simulink model "system"  (R2015a)
settings: Solver=ode45  StartTime=0.0  StopTime=10.0  RelTol=1e-3
values from neighbouring files (symbols this model uses):
  g = 9.81    [run_sim.m]    (also in run_sim_auto.m; run_sim_test.m; run_sim_test4.m; run_sim_v2.m)
  m = 210    [run_sim_auto.m]    (also in run_sim_test4.m = 150; sim_testing.m; wrkspc_no_1.mat; wrkspc_no_10.mat)
  rho_air = 1.225    [run_sim.m]    (also in run_sim_auto.m; run_sim_test.m; run_sim_test4.m; run_sim_v2.m)
undefined symbols (not defined in the file or in its folder): a, crr
libraries: simulink x1
settings Model: Creator=marco  LastModifiedBy=marco

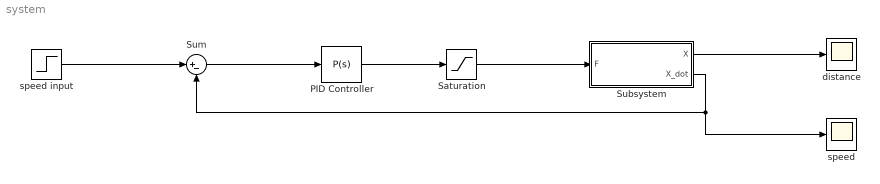
== system system ==
  PID Controller : simulink/Continuous/PID Controller  Controller=P  TimeDomain=Continuous-time  SampleTime=-1  IntegratorMethod=Forward Euler  FilterMethod=Forward Euler  Form=Parallel  UseFilter=on  ControllerParametersSource=internal  P=1  I=0  D=0  N=100  InitialConditionSource=internal  InitialConditionForIntegrator=0  InitialConditionForFilter=0  ExternalReset=none  LimitOutput=off  UpperSaturationLimit=inf  LowerSaturationLimit=-inf  LinearizeAsGain=on  AntiWindupMode=none  Kb=1  TrackingMode=off  Kt=1  PParamMin=[]  PParamMax=[]  IParamMin=[]  IParamMax=[]  DParamMin=[]  DParamMax=[]  NParamMin=[]  NParamMax=[]  KbParamMin=[]  KbParamMax=[]  KtParamMin=[]  KtParamMax=[]  POutMin=[]  POutMax=[]  IOutMin=[]  IOutMax=[]  DOutMin=[]  DOutMax=[]  NOutMin=[]  NOutMax=[]  KbOutMin=[]  KbOutMax=[]  KtOutMin=[]  KtOutMax=[]  IntegratorOutMin=[]  IntegratorOutMax=[]  FilterOutMin=[]  FilterOutMax=[]  SumOutMin=[]  SumOutMax=[]  SumI1OutMin=[]  SumI1OutMax=[]  SumI2OutMin=[]  SumI2OutMax=[]  SumI3OutMin=[]  SumI3OutMax=[]  SumDOutMin=[]  SumDOutMax=[]  SaturationOutMin=[]  SaturationOutMax=[]  IntegratorContinuousStateAttributes=''  IntegratorStateMustResolveToSignalObject=off  IntegratorRTWStateStorageClass=Auto  FilterContinuousStateAttributes=''  FilterStateMustResolveToSignalObject=off  FilterRTWStateStorageClass=Auto  DifferentiatorICPrevScaledInput=0  DifferentiatorOutMin=[]  DifferentiatorOutMax=[]
  Saturation : Saturate
  Subsystem : Subsystem
  Sum : Sum  Inputs=|+-
  distance : Scope
  speed : Scope
  speed input : Step  Before=1  SampleTime=0
  wires:
  Saturation/1 -> Subsystem/1(F)
  PID Controller/1 -> Saturation/1
  Sum/1 -> PID Controller/1
  Subsystem/2(X_dot) -> speed/1, Sum/2
  Subsystem/1(X) -> distance/1
  speed input/1 -> Sum/1

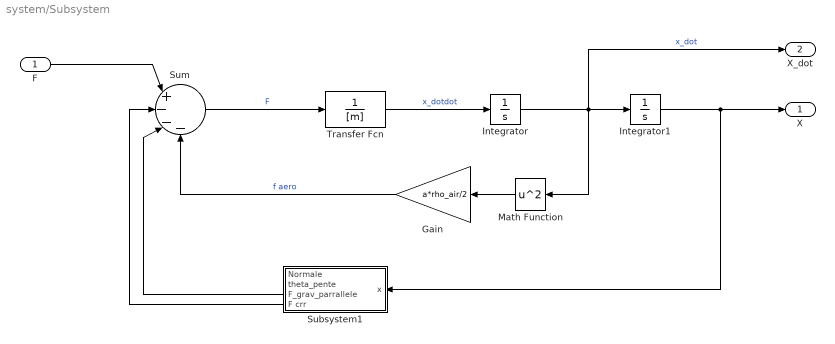
== system system/Subsystem ==
  F : Inport
  Gain : Gain  Gain=a*rho_air/2
  Integrator : Integrator
  Integrator1 : Integrator
  Math Function : Math  Operator=square  SaturateOnIntegerOverflow=on
  Subsystem1 : Subsystem
  Sum : Sum  Inputs=|+---
  Transfer Fcn : TransferFcn  Denominator=[m]
  X : Outport
  X_dot : Outport  Port=2
  wires:
  Sum/1 -> Transfer Fcn/1  "F"
  Transfer Fcn/1 -> Integrator/1  "x_dotdot"
  Integrator/1 -> Math Function/1, X_dot/1, Integrator1/1  "x_dot"
  Gain/1 -> Sum/4  "f aero"
  F/1 -> Sum/1
  Integrator1/1 -> Subsystem1/1(x), X/1
  Subsystem1/3(F_grav_parrallele) -> Sum/3
  Subsystem1/4(F crr) -> Sum/2
  Math Function/1 -> Gain/1

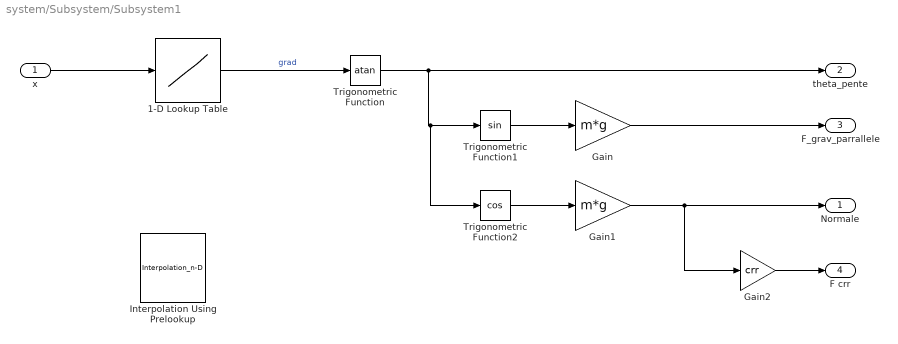
== system system/Subsystem/Subsystem1 ==
  x : Inport
  1-D Lookup Table : Lookup_n-D  NumberOfTableDimensions=1  BreakpointsForDimension1=[-5:5]  Table=tanh([-5:5])  InternalRulePriority=Speed  RndMeth=Simplest  InputSameDT=on
  Gain : Gain  Gain=m*g
  Gain1 : Gain  Gain=m*g
  Gain2 : Gain  Gain=crr
  Interpolation Using Prelookup : Interpolation_n-D  InternalRulePriority=Speed
  Trigonometric Function : Trigonometry  Operator=atan
  Trigonometric Function1 : Trigonometry
  Trigonometric Function2 : Trigonometry  Operator=cos
  Normale : Outport
  theta_pente : Outport  Port=2
  F_grav_parrallele : Outport  Port=3
  F crr : Outport  Port=4
  wires:
  x/1 -> 1-D Lookup Table/1
  1-D Lookup Table/1 -> Trigonometric Function/1  "grad"
  Trigonometric Function/1 -> Trigonometric Function2/1, Trigonometric Function1/1, theta_pente/1
  Trigonometric Function1/1 -> Gain/1
  Trigonometric Function2/1 -> Gain1/1
  Gain1/1 -> Gain2/1, Normale/1
  Gain/1 -> F_grav_parrallele/1
  Gain2/1 -> F crr/1
